simulink model "PistonModelComparison"  (R2020b)
settings: Solver=VariableStepAuto  StartTime=0.0  StopTime=400  RelTol=1e-3
values from neighbouring files (symbols this model uses):
  botA = 0.0378    [ComparisonScript.m]
  pistonStroke = 10    [ComparisonScript.m]
  topA = 0.0378    [ComparisonScript.m]
undefined symbols (not defined in the file or in its folder): PistonHighPressureOriginal, PistonLowPressureOriginal, PistonVelocityOriginal
libraries: fl_lib x12, nesl_utility x9, sh_lib x1
settings Model: Creator=jleonqu  LastModifiedBy=jleonqu

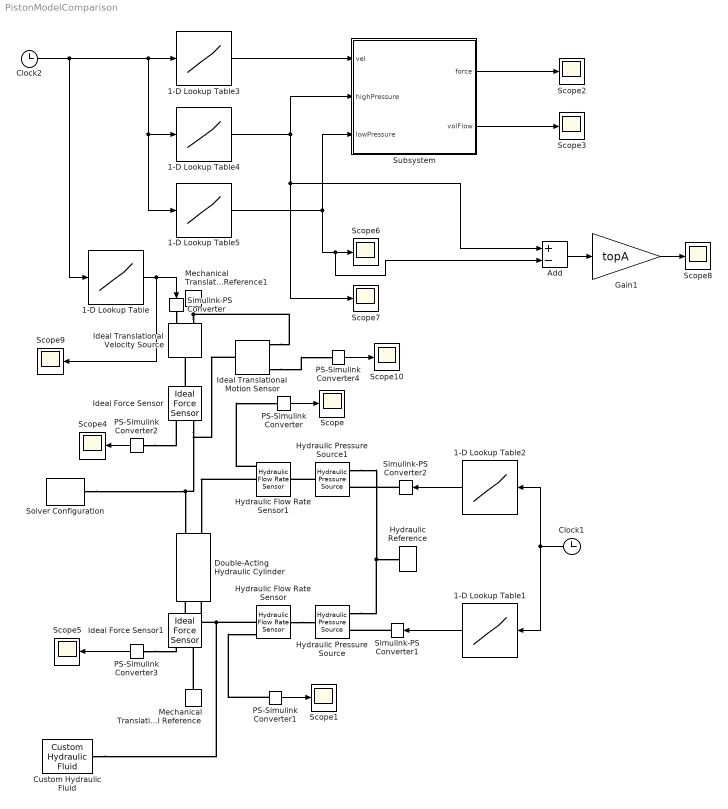
== system PistonModelComparison ==
  1-D Lookup Table : Lookup_n-D  NumberOfTableDimensions=1  BreakpointsForDimension1=PistonVelocityOriginal(:,1)  Table=PistonVelocityOriginal(:,2)  InternalRulePriority=Speed  RndMeth=Simplest  InputSameDT=on
  1-D Lookup Table1 : Lookup_n-D  NumberOfTableDimensions=1  BreakpointsForDimension1=PistonLowPressureOriginal(:,1)  Table=PistonLowPressureOriginal(:,2)  InternalRulePriority=Speed  RndMeth=Simplest  InputSameDT=on
  1-D Lookup Table2 : Lookup_n-D  NumberOfTableDimensions=1  BreakpointsForDimension1=PistonHighPressureOriginal(:,1)  Table=PistonHighPressureOriginal(:,2)  InternalRulePriority=Speed  RndMeth=Simplest  InputSameDT=on
  1-D Lookup Table3 : Lookup_n-D  NumberOfTableDimensions=1  BreakpointsForDimension1=PistonVelocityOriginal(:,1)  Table=PistonVelocityOriginal(:,2)  InternalRulePriority=Speed  RndMeth=Simplest  InputSameDT=on
  1-D Lookup Table4 : Lookup_n-D  NumberOfTableDimensions=1  BreakpointsForDimension1=PistonHighPressureOriginal(:,1)  Table=PistonHighPressureOriginal(:,2)  InternalRulePriority=Speed  RndMeth=Simplest  InputSameDT=on
  1-D Lookup Table5 : Lookup_n-D  NumberOfTableDimensions=1  BreakpointsForDimension1=PistonLowPressureOriginal(:,1)  Table=PistonLowPressureOriginal(:,2)  InternalRulePriority=Speed  RndMeth=Simplest  InputSameDT=on
  Add : Sum  Inputs=+-
  Clock1 : Clock
  Clock2 : Clock
  Custom Hydraulic Fluid : fl_lib/Hydraulic/Hydraulic Utilities/Custom Hydraulic Fluid  density=850 kg/m^3  viscosity_kin=18e-6 m^2/s  bulk=0.8e9*100 Pa  alpha=0.00005  range_error=2
      settings: SourceProductBaseCode=SS  InternalSimscapePortConfiguration="{\"Bottom\":[],\"Left\":[],\"Right\":[{\"id\":\"G\",\"label\":\"\",\"type\":\"foundation.hydraulic.hydraulic\"}],\"Top\":[]}"
  Double-Acting Hydraulic Cylinder : sh_lib/Hydraulic Cylinders/Double-Acting Hydraulic Cylinder  area_A=topA m^2  area_B=botA m^2  stroke=pistonStroke m  init_pos=0.2*pistonStroke m  dead_vol_A=1e-4 m^3  dead_vol_B=1e-4 m^3  init_pressure_A=0 Pa  init_pressure_B=0 Pa  k_sh=1.4  stiff=1e6 N/m  D=150 N/(m/s)  hardstop_model=1  transition=0.1 mm  or=1
      settings: SourceProductBaseCode=SH  InternalSimscapePortConfiguration="{\"Bottom\":[],\"Left\":[{\"id\":\"C\",\"label\":\"C\",\"type\":\"foundation.mechanical.translational.translational\"},{\"id\":\"A\",\"label\":\"A\",\"type\":\"foundation.hydraulic.hydraulic\"}],\"Right\":[{\"id\":\"R\",\"label\":\"R\",\"type\":\"foundation.mechanical.translational.translational\"},{\"id\":\"B\",\"label\":\"B\",\"type\":\"foundation.hydraulic.hydraulic\"}],\"Top\":[]}"
  Gain1 : Gain  Gain=topA
  Hydraulic Flow Rate Sensor : fl_lib/Hydraulic/Hydraulic Sensors/Hydraulic Flow Rate Sensor
  Hydraulic Flow Rate Sensor1 : fl_lib/Hydraulic/Hydraulic Sensors/Hydraulic Flow Rate Sensor
  Hydraulic Pressure Source : fl_lib/Hydraulic/Hydraulic Sources/Hydraulic Pressure Source
      settings: SourceProductBaseCode=SS  InternalSimscapePortConfiguration="{\"Bottom\":[],\"Left\":[{\"id\":\"P\",\"label\":\"P\",\"type\":\"foundation.hydraulic.hydraulic\"}],\"Right\":[{\"id\":\"S\",\"label\":\"S\",\"type\":\"input\"},{\"id\":\"T\",\"label\":\"T\",\"type\":\"foundation.hydraulic.hydraulic\"}],\"Top\":[]}"
  Hydraulic Pressure Source1 : fl_lib/Hydraulic/Hydraulic Sources/Hydraulic Pressure Source
      settings: SourceProductBaseCode=SS  InternalSimscapePortConfiguration="{\"Bottom\":[],\"Left\":[{\"id\":\"P\",\"label\":\"P\",\"type\":\"foundation.hydraulic.hydraulic\"}],\"Right\":[{\"id\":\"S\",\"label\":\"S\",\"type\":\"input\"},{\"id\":\"T\",\"label\":\"T\",\"type\":\"foundation.hydraulic.hydraulic\"}],\"Top\":[]}"
  Hydraulic Reference : fl_lib/Hydraulic/Hydraulic Elements/Hydraulic Reference
  Ideal Force Sensor : fl_lib/Mechanical/Mechanical Sensors/Ideal Force Sensor
  Ideal Force Sensor1 : fl_lib/Mechanical/Mechanical Sensors/Ideal Force Sensor
  Ideal Translational Motion Sensor : fl_lib/Mechanical/Mechanical Sensors/Ideal Translational Motion Sensor  offset=0 m
  Ideal Translational Velocity Source : fl_lib/Mechanical/Mechanical Sources/Ideal Translational Velocity Source
  Mechanical Translational Reference : fl_lib/Mechanical/Translational Elements/Mechanical Translational Reference
  Mechanical Translational Reference1 : fl_lib/Mechanical/Translational Elements/Mechanical Translational Reference
  PS-Simulink Converter{,1..4} (5 alike) : nesl_utility/PS-Simulink Converter  PhysicalDomain=network_engine_domain  SubClassName=ps_output  LeftPortType=input  RightPortType=output  PseudoPeriodic=off  Frequencies=[]  Unit=inherit  AffineConversion=off
  Scope{,1..10} (11 alike) : Scope
  Simulink-PS Converter : nesl_utility/Simulink-PS Converter  PhysicalDomain=network_engine_domain  SubClassName=ps_input  LeftPortType=input  RightPortType=output  PseudoPeriodic=off  Frequencies=[]  NoiseDistribution=none  NoiseParameters=[]  Unit=1  AffineConversion=off  FilteringAndDerivatives=provide  SimscapeFilterOrder=1  InputFilterTimeConstant=0.001  UdotUserProvided=0
  Simulink-PS Converter1 : nesl_utility/Simulink-PS Converter  PhysicalDomain=network_engine_domain  SubClassName=ps_input  LeftPortType=input  RightPortType=output  PseudoPeriodic=off  Frequencies=[]  NoiseDistribution=none  NoiseParameters=[]  Unit=1  AffineConversion=off  FilteringAndDerivatives=provide  SimscapeFilterOrder=1  InputFilterTimeConstant=0.001  UdotUserProvided=0
  Simulink-PS Converter2 : nesl_utility/Simulink-PS Converter  PhysicalDomain=network_engine_domain  SubClassName=ps_input  LeftPortType=input  RightPortType=output  PseudoPeriodic=off  Frequencies=[]  NoiseDistribution=none  NoiseParameters=[]  Unit=1  AffineConversion=off  FilteringAndDerivatives=provide  SimscapeFilterOrder=1  InputFilterTimeConstant=0.001  UdotUserProvided=0
  Solver Configuration : nesl_utility/Solver Configuration  PhysicalDomain=network_engine_domain  SubClassName=solver  LeftPortType=input  RightPortType=generic  Tones=[]  Harmonics=[]  SimulateNoise=off  Profile=off  UseLocalSampling=off  EnableSwitchedLinearOptims=on  FrequencyDomain=off  UseCCode=off  RelTol=0.001  AbsTol=1e-06  MinStep=1e-09  ToWorkspace=off  RevertToSquareIcSolve=off  NumHomotopyIterations=100  PhasorMode=off  PhasorModeNumHarmonics=1  DoDC=off  ResidualTolerance=1e-09  UseLocalSolver=on  LocalSolverChoice=NE_BACKWARD_EULER_ADVANCER  LocalSolverSampleTime=0.001  DoFixedCost=on  MaxNonlinIter=3  MaxModeIter=2  ComputeImpulses=off  ImpulseIterations=2  LinearAlgebra=auto  EquationFormulation=NE_TIME_EF  DelaysMemoryBudget=1024  AutomaticFiltering=on  FilteringTimeConstant=0.001  PartitionStorageMethod=AS_NEEDED  PartitionMemoryBudget=1024  PartitionMethod=ROBUST
  Subsystem : Subsystem
  wires:
  1-D Lookup Table/1 -> Scope9/1, Simulink-PS Converter/1
  Clock2/1 -> 1-D Lookup Table5/1, 1-D Lookup Table4/1, 1-D Lookup Table3/1, 1-D Lookup Table/1
  1-D Lookup Table1/1 -> Simulink-PS Converter1/1
  1-D Lookup Table2/1 -> Simulink-PS Converter2/1
  Clock1/1 -> 1-D Lookup Table2/1, 1-D Lookup Table1/1
  PS-Simulink Converter/1 -> Scope/1
  PS-Simulink Converter1/1 -> Scope1/1
  1-D Lookup Table3/1 -> Subsystem/1(vel)
  1-D Lookup Table5/1 -> Add/2, Scope6/1, Subsystem/3(lowPressure)
  Subsystem/1(force) -> Scope2/1
  Subsystem/2(volFlow) -> Scope3/1
  PS-Simulink Converter2/1 -> Scope4/1
  PS-Simulink Converter3/1 -> Scope5/1
  1-D Lookup Table4/1 -> Add/1, Scope7/1, Subsystem/2(highPressure)
  Add/1 -> Gain1/1
  Gain1/1 -> Scope8/1
  PS-Simulink Converter4/1 -> Scope10/1
  connections:
  Solver Configuration/RConn1 -- Ideal Translational Motion Sensor/LConn1 -- Ideal Force Sensor/RConn1 -- Double-Acting Hydraulic Cylinder/RConn1
  Mechanical Translational Reference1/LConn1 -- Ideal Translational Motion Sensor/RConn1 -- Ideal Translational Velocity Source/RConn2
  Simulink-PS Converter/RConn1 -- Ideal Translational Velocity Source/RConn1
  Simulink-PS Converter1/RConn1 -- Hydraulic Pressure Source/RConn1
  Simulink-PS Converter2/RConn1 -- Hydraulic Pressure Source1/RConn1
  Hydraulic Pressure Source/RConn2 -- Hydraulic Pressure Source1/RConn2 -- Hydraulic Reference/LConn1
  Hydraulic Flow Rate Sensor/LConn1 -- Hydraulic Pressure Source/LConn1
  Hydraulic Flow Rate Sensor/RConn2 -- Custom Hydraulic Fluid/RConn1 -- Double-Acting Hydraulic Cylinder/LConn2
  Hydraulic Pressure Source1/LConn1 -- Hydraulic Flow Rate Sensor1/LConn1
  Hydraulic Flow Rate Sensor1/RConn2 -- Double-Acting Hydraulic Cylinder/RConn2
  Hydraulic Flow Rate Sensor1/RConn1 -- PS-Simulink Converter/LConn1
  PS-Simulink Converter1/LConn1 -- Hydraulic Flow Rate Sensor/RConn1
  Ideal Force Sensor/LConn1 -- Ideal Translational Velocity Source/LConn1
  PS-Simulink Converter2/LConn1 -- Ideal Force Sensor/RConn2
  Ideal Force Sensor1/LConn1 -- Double-Acting Hydraulic Cylinder/LConn1
  Mechanical Translational Reference/LConn1 -- Ideal Force Sensor1/RConn1
  PS-Simulink Converter3/LConn1 -- Ideal Force Sensor1/RConn2
  Ideal Translational Motion Sensor/RConn3 -- PS-Simulink Converter4/LConn1

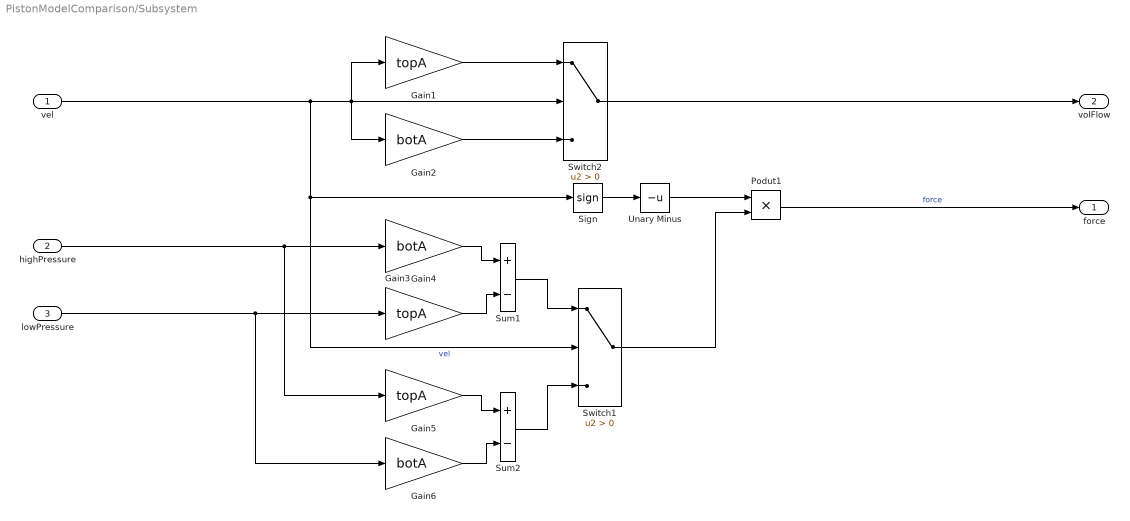
== system PistonModelComparison/Subsystem ==
  vel : Inport
  highPressure : Inport  Port=2
  lowPressure : Inport  Port=3
  Gain1 : Gain  Gain=topA
  Gain2 : Gain  Gain=botA
  Gain3 : Gain  Gain=topA
  Gain4 : Gain  Gain=botA
  Gain5 : Gain  Gain=topA
  Gain6 : Gain  Gain=botA
  Podut1 : Product  RndMeth=Zero
  Sign : Signum
  Sum1 : Sum  Inputs=+-
  Sum2 : Sum  Inputs=+-
  Switch1 : Switch  Criteria=u2 > Threshold
  Switch2 : Switch  Criteria=u2 > Threshold
  Unary Minus : UnaryMinus
  force : Outport
  volFlow : Outport  Port=2
  wires:
  Gain4/1 -> Sum1/1
  lowPressure/1 -> Gain3/1, Gain6/1
  Switch2/1 -> volFlow/1
  Sign/1 -> Unary Minus/1
  Unary Minus/1 -> Podut1/1
  Switch1/1 -> Podut1/2
  vel/1 -> Gain1/1, Switch2/2, Gain2/1, Sign/1, Switch1/2  "vel"
  Gain1/1 -> Switch2/1
  highPressure/1 -> Gain4/1, Gain5/1
  Gain5/1 -> Sum2/1
  Gain3/1 -> Sum1/2
  Podut1/1 -> force/1  "force"
  Gain2/1 -> Switch2/3
  Sum1/1 -> Switch1/1
  Sum2/1 -> Switch1/3
  Gain6/1 -> Sum2/2
